simulink model "Green_H2_Solar_Only"  (R2025a)
settings: Solver=daessc  StartTime=0.0  StopTime=3600*3  MaxStep=60/10  RelTol=1e-3  AbsTol=1e-3
values from neighbouring files (symbols this model uses):
  DH = 285.8e3    (= 285800)    [Parameter_File.m]
  dT_setpoint = 8    [Parameter_File.m]
  R_h2 = 4.12    [Hydrogen_Prop_File.m]
  TDS = 48.7e3    (= 48700)    [Parameter_File.m]
undefined symbols (not defined in the file or in its folder): Control, Electric, Plate, Solar
libraries: fl_lib x26, nesl_utility x13, ee_lib x3
(part 4 of 4)

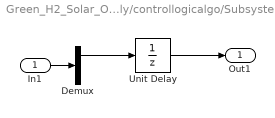
== system Green_H2_Solar_Only/controllogicalgo/Subsystem3 ==
  In1 : Inport
  Demux : Demux  Outputs=2
  Unit Delay : UnitDelay  SampleTime=60  HasFrameUpgradeWarning=on
  Out1 : Outport
  wires:
  Demux/1 -> Unit Delay/1
  In1/1 -> Demux/1
  Unit Delay/1 -> Out1/1

== matlab function Green_H2_Solar_Only/controllogicalgo/MATLAB Function ==
  data: u input; y output; theta input; dtheta input; Re input
function y = fcn(u, theta, dtheta, Re)
DH = u(1); TDS = u(2);
G0 = DH-((theta-dtheta)/298)*TDS;
y = sqrt(G0*Re);

== matlab function Green_H2_Solar_Only/Sensor/MATLAB Function ==
  data: u input; Z output
function Z = fcn(u)

Z = min(u(2)/u(1),1e3);
